simulink model "uz_codegen"  (R2021a)
settings: Solver=VariableStepAuto  StartTime=0.0  StopTime=0.5  RelTol=1e-3  EnableMultiTasking=on
PreLoadFcn:
  | uz_setCodegenPaths
model workspace (MATLAB code in the model file):
  | cmdLim = Simulink.Parameter;
  | cmdLim.Value = 15;
  | cmdLim.Description = 'Limit for controlling the maximum surface command angle.';
  | cmdLim.Min = 0;
  | cmdLim.Max = 90;
  | cmdLim.DocUnits = 'deg';
  | 
  | dispGain = Simulink.Parameter;
  | dispGain.Value = 0.75;
  | dispGain.Description = 'Gain applied to the displacement error.';
  | dispGain.Min = 0;
  | dispGain.Max = [];
  | dispGain.DocUnits = 'deg/sec/deg';
  | 
  | dispLim = Simulink.Parameter;
  | dispLim.Value = 30;
  | dispLim.Description = 'Limit for controlling the maximum commanded angle.';
  | dispLim.Min = 0;
  | dispLim.Max = 180;
  | dispLim.DocUnits = 'deg';
  | 
  | intGain = Simulink.Parameter;
  | intGain.Value = 0.5;
  | intGain.Description = 'Gain applied to the integral error.';
  | intGain.Min = 0;
  | intGain.Max = [];
  | intGain.DocUnits = 'deg/sec/deg/sec';
  | 
  | intLim = Simulink.Parameter;
  | intLim.Value = 5;
  | intLim.Description = 'Limit for controlling the maximum commanded angle.';
  | intLim.Min = 0;
  | intLim.Max = 90;
  | intLim.DocUnits = 'deg';
  | 
  | rateGain = Simulink.Parameter;
  | rateGain.Value = 2;
  | rateGain.Description = 'Gain applied to the rate error.';
  | rateGain.Min = 0;
  | rateGain.Max = [];
  | rateGain.DocUnits = 'deg/deg/sec';
  | 
  | rateLim = Simulink.Parameter;
  | rateLim.Value = 6;
  | rateLim.Description = 'Limit for controlling the maximum commanded angle.';
  | rateLim.Min = 0;
  | rateLim.Max = 180;
  | rateLim.DocUnits = 'deg/sec';
  | 
  | hdgGain = Simulink.Parameter;
  | hdgGain.Value = 0.015;
values from neighbouring files (symbols this model uses):
  f_switchingInverter = 10000    [PMSM_01_Parameter.m]
  I_max = 50    [PMSM_01_Parameter.m]
  Ki_IdController = Kp_IdController * Ki_IdController    (= 100.530964915)    [PMSM_01_Parameter.m]
  Ki_IqController = Kp_IqController * Ki_IqController    (= 100.530964915)    [PMSM_01_Parameter.m]
  Ki_SpeedController = Kp_SpeedController * Ki_SpeedController    (= 50.6340660401)    [PMSM_01_Parameter.m]
  Kp_IdController = Kp_IdController    (= 0.0402123859659)    [PMSM_01_Parameter.m]
  Kp_IqController = Kp_IqController    (= 0.0402123859659)    [PMSM_01_Parameter.m]
  Kp_SpeedController = Kp_SpeedController    (= 0.725279570921)    [PMSM_01_Parameter.m]
  Ld = Lq    (= 1.6e-05)    [PMSM_01_Parameter.m]
  Lq = 16e-6    (= 1.6e-05)    [PMSM_01_Parameter.m]
  psi_pm = 0.0048    [PMSM_01_Parameter.m]
  T_controller = 1/f_CurrentController    (= 5e-05)    [PMSM_01_Parameter.m]
  T_dead = 2e-6    (= 2e-06)    [PMSM_01_Parameter.m]
  U_DC = 46    [PMSM_01_Parameter.m]
  zp = 21    [PMSM_01_Parameter.m]
undefined symbols (not defined in the file or in its folder): DiscIntNeverNeededParam, U_maxDQ
libraries: nesl_utility x17, ee_lib x15, fl_lib x13, simulink x7, pid_lib x3, dspsrcs4 x3, spsTriangleGeneratorLib x1, spsabctodq0Lib x1, spsdq0toabcLib x1, spsdq0toAlphaBetaZeroLib x1, embmathops x1
(part 1 of 2)
settings Model: RequirementInfo={} %GIDa_fe9045fd_0412_4b6e_8206_617cc20e6fde  FPTRunName=Active  Creator=ts  LastModifiedBy=wilflingti66489
settings SolverCC: AlgebraicLoopSolver=TrustRegion  PositivePriorityOrder=on  AutoInsertRateTranBlk=on
settings DataIOCC: SaveOutput=off  SignalLogging=off  DSMLogging=off  SaveTime=off
settings OptimizationCC: DefaultParameterBehavior=Inlined  UseDivisionForNetSlopeComputation=on  GainParamInheritBuiltInType=on  UseFloatMulNetSlope=on  DefaultUnderspecifiedDataType=single  UseSpecifiedMinMax=on  InlineInvariantSignals=on  PassReuseOutputArgsAs=Individual arguments  NoFixptDivByZeroProtection=on  EfficientFloat2IntCast=on  LifeSpan=1  MaxStackSize=64  OptimizeBlockOrder=speed  DifferentSizesBufferReuse=on  EfficientTunableParamExpr=on
settings DebuggingCC: AllowSymbolicDim=off  SFUnexpectedBacktrackingDiag=warning  SFNoUnconditionalDefaultTransitionDiag=warning  SFExecutionAtInitializationDiag=none  SFMachineParentedDataDiag=warning  ArithmeticOperatorsInVariantConditions=warning
settings HardwareCC: ProdBitPerPointer=32  ProdBitPerSizeT=32  ProdBitPerPtrDiffT=32  ProdLargestAtomicInteger=Long  ProdLargestAtomicFloat=Double  ProdWordSize=32  ProdLongLongMode=on  ProdHWDeviceType=ARM Compatible->ARM Cortex-R  HardwareBoardFeatureSet=SoCBlockset
settings SFSimCC: MATLABDynamicMemAlloc=off
settings RTWCC: SystemTargetFile=ert.tlc  GenCodeOnly=on  TemplateMakefile=ert_default_tmf  GenerateReport=on  BuildConfiguration=Faster Runs  IncludeHyperlinkInReport=on  GenerateCodeMetricsReport=on  CheckMdlBeforeBuild=Warning
settings CodeAppCC: ForceParamTrailComments=on  IgnoreCustomStorageClasses=off  OperatorAnnotations=on  SimulinkDataObjDesc=on  SFDataObjDesc=on  MATLABFcnDesc=on  CustomSymbolStrGlobalVar=rt$N$M  CustomSymbolStrType=$N$M  CustomSymbolStrFcn=$N$M$F  CustomSymbolStrMacro=$N$M  InsertBlockDesc=on  StateflowObjectComments=on  MATLABSourceComments=on  EnableCustomComments=on  ReqsInCode=on
settings ERTTargetCC: TargetLangStandard=C99 (ISO)  CodeReplacementLibrary=GNU C99 extensions  MultiwordLength=2048  IncludeMdlTerminateFcn=off  CombineSignalStateStructs=on  SuppressErrorStatus=on  IncludeFileDelimiter=UseQuote  CodeInterfacePackaging=Reusable function  RemoveResetFunc=off  InlinedParameterPlacement=NonHierarchical  MultiInstanceErrorCode=Warning  RootIOFormat=Part of model data structure  ERTCustomFileTemplate=example_file_process.tlc  GlobalDataDefinition=InSourceFile  GlobalDataReference=InSourceFile  ERTFilePackagingFormat=CompactWithDataFile
settings ConfigComp: CovScope=ReferencedModels  CovSaveName=covdata_rollAP  CovMetricSettings=dcmtrwe  CovHTMLOptions=-sRT=1 -aTS=1 -bRG=1 -bTC=1 -hTR=1 -nFC=0 -scm=1 -bcm=1 -xEv=0  CovSaveCumulativeToWorkspaceVar=on  CovSaveSingleToWorkspaceVar=on  CovCumulativeVarName=covCumulativeData_rollAP  CovReportOnPause=off  CovExternalEMLEnable=off  CovSFcnEnable=off

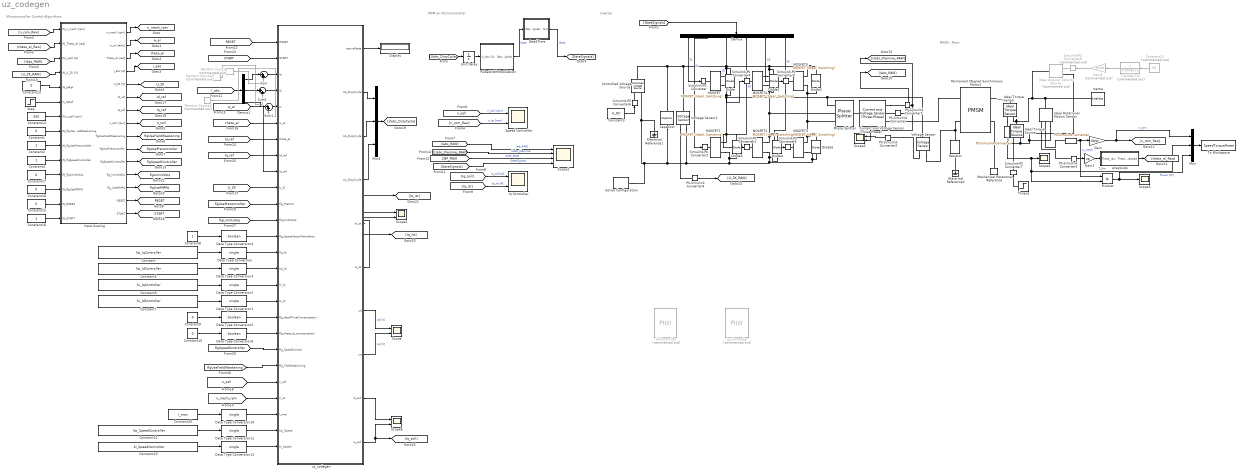
== system uz_codegen ==
  note: Inverter
  note: PWM on Microcontroller
  note: PMSM - Plant
  note: Microcontroller Control-Algorithms
  " " : nesl_utility/PS-Simulink Converter  PhysicalDomain=network_engine_domain  SubClassName=ps_output  LeftPortType=input  RightPortType=output  PseudoPeriodic=off  Frequencies=[]  Unit=inherit  AffineConversion=off
      settings: SourceProductBaseCode=PW,SS
  " 1" : nesl_utility/PS-Simulink Converter  PhysicalDomain=network_engine_domain  SubClassName=ps_output  LeftPortType=input  RightPortType=output  PseudoPeriodic=off  Frequencies=[]  Unit=inherit  AffineConversion=off
      settings: SourceProductBaseCode=PW,SS
  Capacitor : fl_lib/Electrical/Electrical Elements/Capacitor  c=Capacitance_CircuitCondensator uF  r=1e-6 Ohm  g=0 1/Ohm  i_specify=off  i_priority=None  i=0 A  i_nominal_specify=off  i_nominal_unit=A  i_nominal_value=1  v_specify=off  v_priority=None  v=0 V  v_nominal_specify=off  v_nominal_unit=V  v_nominal_value=1  vc_specify=off  vc_priority=High  vc=0 V  vc_nominal_specify=off  vc_nominal_unit=V  vc_nominal_value=1
  Constant : Constant  Value=Kp_IqController
  Constant{1,9..10,13,15,17..18} (7 alike) : Constant  Value=0
  Constant12 : Constant  Commented=on  Value=50
  Constant14 : Constant  Value=500
  Constant{2,4,8,16} (4 alike) : Constant
  Constant20 : Constant  Value=I_max
  Constant22 : Constant  Value=Kp_SpeedController
  Constant23 : Constant  Value=Ki_SpeedController
  Constant3 : Constant  Value=U_DC
  Constant5 : Constant  Value=Kp_IdController
  Constant6 : Constant  Value=Ki_IqController
  Constant7 : Constant  Value=Ki_IdController
  Controlled Voltage Source : fl_lib/Electrical/Electrical Sources/Controlled Voltage Source
  Current and Voltage Sensor (Three-Phase) : ee_lib/Sensors & Transducers/Current and Voltage Sensor (Three-Phase)  vMeasurementType=ee.enum.vmeasurement.ll  outputUnit=ee.enum.unit.si  SRated=100e6 V*A  VRated=24e3 V  I_specify=off  I_priority=None  I=[ 0 0 0 ] A  I_nominal_specify=off  I_nominal_unit=A  I_nominal_value=1  V_specify=off  V_priority=None  V=[ 0 0 0 ] V  V_nominal_specify=off  V_nominal_unit=V  V_nominal_value=1
      settings: SourceProductBaseCode=PS  InternalSimscapePortConfiguration="{\"Bottom\":[],\"Left\":[{\"id\":\"N1\",\"label\":\"~1\",\"type\":\"foundation.electrical.three_phase\"}],\"Right\":[{\"id\":\"V_output\",\"label\":\"V\",\"type\":\"output\"},{\"id\":\"I_output\",\"label\":\"I\",\"type\":\"output\"},{\"id\":\"N2\",\"label\":\"~2\",\"type\":\"foundation.electrical.three_phase\"}],\"Top\":[]}"
  Data Type Conversion{,1..3,10..12} (7 alike) : DataTypeConversion  OutDataTypeStr=single
  Data Type Conversion4 : DataTypeConversion  OutDataTypeStr=boolean
  Data Type Conversion5 : DataTypeConversion  OutDataTypeStr=boolean
  Data Type Conversion6 : DataTypeConversion  OutDataTypeStr=boolean
  DeadTime : Subsystem
  Demux : Demux  Outputs=6
  Demux1 : Demux  Outputs=3
  Diode{,1..5} (6 alike) : ee_lib/Semiconductors & Converters/Diode  ModelType=ee.enum.diode.modelType.pwl  IfMat=[.07, .12, .19, 1.75, 4.24, 7.32, 11.2; .16, .3, .72, 2.14, 4.02, 6.35, 9.12] A  TjVec=[25, 125] degC  VfVec=[.5, .7, .9, 1.3, 1.7, 2.1, 2.5] V  Vf=0.1 V  Ron=0.001 Ohm  Goff=1e-5 1/Ohm  prmExp=ee.enum.diode.expParam.useTwo  I12=[.0137, .545] A  V12=[.6, .7] V  IS=1e-12 A  ec=1  I1=0.0137 A  V1=0.6 V  RS=0 Ohm  Tmeas=25 degC  N_series=1  N_parallel=1  Rz=0.3 Ohm  BV=inf V  C_param=ee.enum.diode.capParam.fixed  CJ=0 pF  CJ0=5 pF  VJ=1 V  Mgrad=0.5  Vvec=[.1, 10, 100] V  Cvec=[3.5, 1, .4] pF  FC=0.5  Q_param=ee.enum.diode.recoveryParam.off  iRM=-7.15 A  iF=4 A  didt=-750 A/us  trr_factor=3  trr=115 ns  Qrr=1500 s*uA  TT=50 ns  tau=100 ns  T_param=ee.enum.diode.temperatureParam.off  IS_T2=1.25e-7 A  I1_T2=0.245 A  V1_T2=0.5 V  Tmeas2=125 degC  EG_param=ee.enum.diode.egapParam.material_si  EG=1.11 eV  XTI_param=ee.enum.diode.xtiParam.pn  XTI=3  dBVdT=0 V/K  enable_faults=ee.enum.faults.faultEnable.no  fault_action=ee.enum.faults.faultAction.none  fault_types=ee.enum.diode.faults.open  tau_fault=1e-3 s  IfMat_faulted=[.07, .12, .19, 1.75, 4.24, 7.32, 11.2; .16, .3, .72, 2.14, 4.02, 6.35, 9.12] A  VfVec_faulted=[.5, .7, .9, 1.3, 1.7, 2.1, 2.5] V  Ropen_faulted=1000 Ohm  Gshort_faulted=1000 1/Ohm  Vf_faulted=0.6 V  Ron_faulted=0.3 Ohm  Goff_faulted=1e-8 S  I12_faulted=[.0137, .545] A  V12_faulted=[.6, .7] V  IS_faulted=1e-12 A  ec_faulted=1  I1_faulted=0.0137 A  V1_faulted=0.6 V  RS_faulted=0 Ohm  Rz_faulted=0.3 Ohm  BV_faulted=inf V  Cscale_faulted=100  enable_temporal_fault=ee.enum.faults.faultEnable.no  t_fault=inf s  enable_behavioral_fault=ee.enum.faults.faultEnable.no  max_permissible_voltage=inf V  n_fail_on_voltage=1  max_permissible_current=inf A  t_fail_on_current=1 s  max_permissible_dVdt=inf V/s  Tdevice=25 degC  i_specify=off  i_priority=None  i=0 A  i_nominal_specify=off  i_nominal_unit=A  i_nominal_value=1  v_specify=off  v_priority=None  v=0 V  v_nominal_specify=off  v_nominal_unit=V  v_nominal_value=1  i_diode_specify=off  i_diode_priority=None  i_diode=0 A  i_diode_nominal_specify=off  i_diode_nominal_unit=A  i_diode_nominal_value=1  v_diode_specify=off  v_diode_priority=None  v_diode=0 V  v_diode_nominal_specify=off  v_diode_nominal_unit=V  v_diode_nominal_value=1  i_capacitor_specify=off  i_capacitor_priority=None  i_capacitor=0 A  i_capacitor_nominal_specify=off  i_capacitor_nominal_unit=A  i_capacitor_nominal_value=1  v_capacitor_specify=off  v_capacitor_priority=None  v_capacitor=0 V  v_capacitor_nominal_specify=off  v_capacitor_nominal_unit=V  v_capacitor_nominal_value=1  power_dissipated_specify=off  power_dissipated_priority=None  power_dissipated=0 W  power_dissipated_nominal_specify=off  power_dissipated_nominal_unit=W  power_dissipated_nominal_value=1  max_permissible_temperature=inf K  t_fail_on_temperature=1 s  thermal_network_parameterization=ee.enum.thermalNetworkTopology.cauer  Rth=[0, 10] K/W  Rth_Foster=[4, 6] K/W  thermal_mass_parameterization=ee.enum.thermalNetwork.timeconstant  thermal_mass=[0, 1] J/K  thermal_mass_Foster=[1.5, 3] J/K  thermal_time_constant=[0, 10] s  thermal_time_constant_Foster=[6, 18] s  thermal_mass_initial_temperatures=[25, 25] degC
  Display : Display
  Electrical Reference1 : fl_lib/Electrical/Electrical Elements/Electrical Reference
  Electrical Reference2 : fl_lib/Electrical/Electrical Elements/Electrical Reference
  Gain : Gain  Gain=30/pi
  Gain1 : Gain  Gain=zp
  Gain2 : Gain  Commented=on  Gain=pi/30
  Id-Controller : pid_lib/PID Controller  Commented=on  Controller=PI  Form=Parallel  TimeDomain=Discrete-time  UseExternalTs=off  SampleTime=-1  IntegratorMethod=Forward Euler  FilterMethod=Forward Euler  ControllerParametersSource=external  P=Kp_IqController  I=Ki_IqController  D=0  UseFilter=on  N=100  TunerSelectOption=Transfer Function Based (PID Tuner App)  InitialConditionSource=internal  InitialConditionForIntegrator=0  InitialConditionForFilter=0  DifferentiatorICPrevScaledInput=0  ExternalReset=level  TrackingMode=off  Kt=1  LimitOutput=on  SatLimitsSource=external  UpperSaturationLimit=U_maxDQ  LowerSaturationLimit=-U_maxDQ  LinearizeAsGain=on  AntiWindupMode=none  Kb=1  POutMin=[]  POutMax=[]  IOutMin=[]  IOutMax=[]  DOutMin=[]  DOutMax=[]  NOutMin=[]  NOutMax=[]  SumOutMin=[]  SumOutMax=[]  SaturationOutMin=[]  SaturationOutMax=[]  PParamMin=[]  PParamMax=[]  IParamMin=[]  IParamMax=[]  DParamMin=[]  DParamMax=[]  NParamMin=[]  NParamMax=[]  KbParamMin=[]  KbParamMax=[]  KtParamMin=[]  KtParamMax=[]  KbOutMin=[]  KbOutMax=[]  KtOutMin=[]  KtOutMax=[]  IntegratorOutMin=[]  IntegratorOutMax=[]  FilterOutMin=[]  FilterOutMax=[]  SumI1OutMin=[]  SumI1OutMax=[]  SumI2OutMin=[]  SumI2OutMax=[]  SumI3OutMin=[]  SumI3OutMax=[]  SumI4OutMin=[]  SumI4OutMax=[]  SumDOutMin=[]  SumDOutMax=[]  DifferentiatorOutMin=[]  DifferentiatorOutMax=[]  FilterDiffOutCoefMin=[]  FilterDiffOutCoefMax=[]  ReciprocalOutMin=[]  ReciprocalOutMax=[]  SumDenOutMin=[]  SumDenOutMax=[]  SumNumOutMin=[]  SumNumOutMax=[]  DivideOutMin=[]  DivideOutMax=[]  UdiffTsProdOutMin=[]  UdiffTsProdOutMax=[]  NTsProdOutMin=[]  NTsProdOutMax=[]  UintegralTsProdOutMin=[]  UintegralTsProdOutMax=[]  UngainTsProdOutMin=[]  UngainTsProdOutMax=[]  IntegratorContinuousStateAttributes=''  IntegratorStateMustResolveToSignalObject=off  IntegratorRTWStateStorageClass=Auto  FilterContinuousStateAttributes=''  FilterStateMustResolveToSignalObject=off  FilterRTWStateStorageClass=Auto  ParallelPVariant=ExternalParameters  IdealPVariant=Disabled  IVariant=ExternalParameters  DVariant=Disabled  IntegratorVariant=Discrete  SatVariant=External  AWVariant=Passthrough  PCopyVariant=Disabled  TRVariant=Disabled  FdbkBlocksVariant=Forward  IdealPFdbkVariant=Disabled  SatFdbkVariant=Disabled  DerivativeFilterVariant=Disabled  NVariant=Disabled  NCopyVariant=Disabled_SignalSpec  FilterICVariant=Disabled  IntegratorICVariant=InternalICs  ExternalResetVariant=ExternalReset  TRSumVariant=Passthrough  SumFdbkVariant=Disabled  SumVariant=Sum_PI  TsampFilterVariant=InternalTs  TsampNgainVariant=Passthrough  TsampIntegralVariant=Passthrough  ExternalSaturationOutDataTypeStr=Inherit: Same as second input
  Ideal Angular Velocity Source : fl_lib/Mechanical/Mechanical Sources/Ideal Angular Velocity Source  Commented=on
  Ideal Rotational Motion Sensor : fl_lib/Mechanical/Mechanical Sensors/Ideal Rotational Motion Sensor  wrap_angle=simscape.enum.onoff.on  offset=0 rad
  Ideal Torque Sensor : fl_lib/Mechanical/Mechanical Sensors/Ideal Torque Sensor
  Ideal Torque Source : fl_lib/Mechanical/Mechanical Sources/Ideal Torque Source
  Inertia : fl_lib/Mechanical/Rotational Elements/Inertia  inertia=J_M kg*m^2  num_ports=foundation.enum.numPorts2.one  w_specify=off  w_priority=High  w=0 rad/s  w_nominal_specify=off  w_nominal_unit=rad/s  w_nominal_value=1  t_specify=off  t_priority=None  t=0 N*m  t_nominal_specify=off  t_nominal_unit=N*m  t_nominal_value=1
  Input Scaling : Subsystem
  Iq Controller : Scope  NumInputPorts=2
  Iq_Controller : pid_lib/PID Controller  Commented=on  Controller=PI  Form=Parallel  TimeDomain=Discrete-time  UseExternalTs=off  SampleTime=-1  IntegratorMethod=Forward Euler  FilterMethod=Forward Euler  ControllerParametersSource=external  P=Kp_IqController  I=Ki_IqController  D=0  UseFilter=on  N=100  TunerSelectOption=Transfer Function Based (PID Tuner App)  InitialConditionSource=internal  InitialConditionForIntegrator=0  InitialConditionForFilter=0  DifferentiatorICPrevScaledInput=0  ExternalReset=level  TrackingMode=off  Kt=1  LimitOutput=on  SatLimitsSource=external  UpperSaturationLimit=U_maxDQ  LowerSaturationLimit=-U_maxDQ  LinearizeAsGain=on  AntiWindupMode=none  Kb=1  POutMin=[]  POutMax=[]  IOutMin=[]  IOutMax=[]  DOutMin=[]  DOutMax=[]  NOutMin=[]  NOutMax=[]  SumOutMin=[]  SumOutMax=[]  SaturationOutMin=[]  SaturationOutMax=[]  PParamMin=[]  PParamMax=[]  IParamMin=[]  IParamMax=[]  DParamMin=[]  DParamMax=[]  NParamMin=[]  NParamMax=[]  KbParamMin=[]  KbParamMax=[]  KtParamMin=[]  KtParamMax=[]  KbOutMin=[]  KbOutMax=[]  KtOutMin=[]  KtOutMax=[]  IntegratorOutMin=[]  IntegratorOutMax=[]  FilterOutMin=[]  FilterOutMax=[]  SumI1OutMin=[]  SumI1OutMax=[]  SumI2OutMin=[]  SumI2OutMax=[]  SumI3OutMin=[]  SumI3OutMax=[]  SumI4OutMin=[]  SumI4OutMax=[]  SumDOutMin=[]  SumDOutMax=[]  DifferentiatorOutMin=[]  DifferentiatorOutMax=[]  FilterDiffOutCoefMin=[]  FilterDiffOutCoefMax=[]  ReciprocalOutMin=[]  ReciprocalOutMax=[]  SumDenOutMin=[]  SumDenOutMax=[]  SumNumOutMin=[]  SumNumOutMax=[]  DivideOutMin=[]  DivideOutMax=[]  UdiffTsProdOutMin=[]  UdiffTsProdOutMax=[]  NTsProdOutMin=[]  NTsProdOutMax=[]  UintegralTsProdOutMin=[]  UintegralTsProdOutMax=[]  UngainTsProdOutMin=[]  UngainTsProdOutMax=[]  IntegratorContinuousStateAttributes=''  IntegratorStateMustResolveToSignalObject=off  IntegratorRTWStateStorageClass=Auto  FilterContinuousStateAttributes=''  FilterStateMustResolveToSignalObject=off  FilterRTWStateStorageClass=Auto  ParallelPVariant=ExternalParameters  IdealPVariant=Disabled  IVariant=ExternalParameters  DVariant=Disabled  IntegratorVariant=Discrete  SatVariant=External  AWVariant=Passthrough  PCopyVariant=Disabled  TRVariant=Disabled  FdbkBlocksVariant=Forward  IdealPFdbkVariant=Disabled  SatFdbkVariant=Disabled  DerivativeFilterVariant=Disabled  NVariant=Disabled  NCopyVariant=Disabled_SignalSpec  FilterICVariant=Disabled  IntegratorICVariant=InternalICs  ExternalResetVariant=ExternalReset  TRSumVariant=Passthrough  SumFdbkVariant=Disabled  SumVariant=Sum_PI  TsampFilterVariant=InternalTs  TsampNgainVariant=Passthrough  TsampIntegralVariant=Passthrough  ExternalSaturationOutDataTypeStr=Inherit: Same as second input
  MOSFET{,1..5} (6 alike) : ee_lib/Semiconductors & Converters/MOSFET (Ideal, Switching)  Rds=0.040 Ohm  Goff=1e-6 1/Ohm  Vth=0.7 V  diode_param=1  diode_Vf=0.8 V  diode_Ron=0.001 Ohm  diode_Goff=1e-5 1/Ohm  diode_C=5e-8 F  diode_iRM=-235 A  diode_iF=300 A  diode_idot=-50 A/us  diode_trr_param=1  diode_trr_factor=3  diode_trr=15 us  diode_Qrr=1.5e+3 s*uA  thermal_loss_option=ee.enum.converters.thermalLossOption.constantvalues  Von_data=[0, 1.1, 1.3, 1.45, 1.75, 2.25, 2.7; 0, 1, 1.15, 1.35, 1.7, 2.35, 3] V  Eon_data=[0, .29, 1.43, 2.86, 5.71, 13.14, 22.86; 0, .57, 2.63, 5.14, 10.29, 20.57, 30.29] * 1e-3 J  Eoff_data=[0, .21, 1.07, 2.14, 4.29, 9.86, 17.14; 0, .43, 1.97, 3.86, 7.71, 15.43, 22.71] * 1e-3 J  Tj=[298.15, 398.15] K  Iout_data=[0, 10, 50, 100, 200, 400, 600] A  Eon_scalar=22.86e-3 J  Eoff_scalar=17.14e-3 J  Voff=300 V  Iout_scalar=600 A  diodeModelType=ee.enum.converters.diodeModelType.pwl  diode_IfMat=[.07, .12, .19, 1.75, 4.24, 7.32, 11.2; .16, .3, .72, 2.14, 4.02, 6.35, 9.12] A  diode_TjVec=[25, 125] degC  diode_VfVec=[.5, .7, .9, 1.3, 1.7, 2.1, 2.5] V  thermal_network_parameterization=ee.enum.thermalNetworkTopology.external  Rth=[.03, .2] K/W  Rth_Foster=[.03, .2] K/W  thermal_mass_parameterization=ee.enum.thermalNetwork.timeconstant  thermal_mass=[3, 25] J/K  thermal_mass_Foster=[33, 50] J/K  thermal_time_constant=[.1, 5] s  thermal_time_constant_Foster=[1, 10] s  thermal_mass_initial_temperatures=[25, 25] degC  junction_thermal_mass=0.1 J/K  vT_specify=off  vT_priority=None  vT=0 V  vT_nominal_specify=off  vT_nominal_unit=V  vT_nominal_value=1  Qj_specify=off  Qj_priority=None  Qj=0 W  Qj_nominal_specify=off  Qj_nominal_unit=W  Qj_nominal_value=1  junction_temperature_specify=off  junction_temperature_priority=None  junction_temperature=25 degC  junction_temperature_nominal_specify=off  junction_temperature_nominal_unit=degC  junction_temperature_nominal_value=1
  Mechanical Rotational Reference : fl_lib/Mechanical/Rotational Elements/Mechanical Rotational Reference
  Mux : Mux  Inputs=3
  Mux1 : Mux  Inputs=3
  PS-Simulink Converter{,1..4} (5 alike) : nesl_utility/PS-Simulink Converter  PhysicalDomain=network_engine_domain  SubClassName=ps_output  LeftPortType=input  RightPortType=output  PseudoPeriodic=off  Frequencies=[]  Unit=inherit  AffineConversion=off
      settings: SourceProductBaseCode=PW,SS
  Permanent Magnet Synchronous Motor1 : ee_lib/Electromechanical/Permanent Magnet/PMSM  winding_type=ee.enum.statorconnection.wye  machine_param=ee.enum.pmsm.parameterization.constant  nPolePairs=zp  pmflux_param=ee.enum.pmflux.fluxlinkage  pm_flux_linkage=psi_pm Wb  torque_constant=0.18 N*m/A  back_emf_constant=0.07 V/(rad/s)  stator_param=ee.enum.statorparam.LdLqL0  Ld=Ld H  Lq=Lq H  idVec=[-200, 0, 200] A  iqVec=[-200, 0, 200] A  LdMatrix=0.0002 * ones(3, 3) H  LqMatrix=0.0002 * ones(3, 3) H  PmMatrix=0.1 * ones(3, 3) Wb  ktMatrix=0.18 * ones(3, 3) N*m/A  keMatrix=0.18 * ones(3, 3) V/(rad/s)  L0=0.00016 H  Ls=0.0002 H  Lm=-0.00002 H  Ms=0.00002 H  Rs=R Ohm  zero_sequence=ee.enum.park.zerosequence.include  J=0.0 kg*m^2  lam=0 N*m/(rad/s)  axes_param=ee.enum.rotorangle.daxis  i_d_specify=off  i_d_priority=None  i_d=0 A  i_d_nominal_specify=off  i_d_nominal_unit=A  i_d_nominal_value=1  i_q_specify=off  i_q_priority=None  i_q=0 A  i_q_nominal_specify=off  i_q_nominal_unit=A  i_q_nominal_value=1  torque_specify=off  torque_priority=None  torque=0 N*m  torque_nominal_specify=off  torque_nominal_unit=N*m  torque_nominal_value=1  angular_velocity_specify=off  angular_velocity_priority=High  angular_velocity=0 deg/s  angular_velocity_nominal_specify=off  angular_velocity_nominal_unit=rpm  angular_velocity_nominal_value=1  angular_position_specify=off  angular_position_priority=High  angular_position=0 deg  angular_position_nominal_specify=off  angular_position_nominal_unit=deg  angular_position_nominal_value=1  loss_param=ee.enum.ironloss.none  losses_oc=[0, 0, 0] W  losses_sc=[0, 0, 0] W  f_losses=60 Hz  Isc_losses=95 A  Tmeas=298.15 K  alpha=3.93e-3 1/K  alpha_flux=-0.001 1/K  stator_thermal_mass=100 J/K  rotor_thermal_mass=200 J/K  Rm_percent_rotor=90  Rd_percent_rotor=30  temperatureA_specify=off  temperatureA_priority=High  temperatureA=25 degC  temperatureA_nominal_specify=off  temperatureA_nominal_unit=degC  temperatureA_nominal_value=1  temperatureB_specify=off  temperatureB_priority=High  temperatureB=25 degC  temperatureB_nominal_specify=off  temperatureB_nominal_unit=degC  temperatureB_nominal_value=1  temperatureC_specify=off  temperatureC_priority=High  temperatureC=25 degC  temperatureC_nominal_specify=off  temperatureC_nominal_unit=degC  temperatureC_nominal_value=1  temperatureR_specify=off  temperatureR_priority=High  temperatureR=25 degC  temperatureR_nominal_specify=off  temperatureR_nominal_unit=degC  temperatureR_nominal_value=1
      settings: InternalSimscapePortConfiguration="{\"Bottom\":[],\"Left\":[{\"id\":\"N\",\"label\":\"~\",\"type\":\"foundation.electrical.three_phase\"},{\"id\":\"n\",\"label\":\"n\",\"type\":\"foundation.electrical.electrical\"}],\"Right\":[{\"id\":\"R\",\"label\":\"R\",\"type\":\"foundation.mechanical.rotational.rotational\"},{\"id\":\"C\",\"label\":\"C\",\"type\":\"foundation.mechanical.rotational.rotational\"}],\"Top\":[]}"
  Phase Splitter : ee_lib/Connectors & References/Phase Splitter
      settings: SourceProductBaseCode=PS
  Product : Product
  PulseWidthModulation : Subsystem
  Random Source : dspsrcs4/Random Source  Commented=on  SrcType=Uniform  NormMethod=Ziggurat  CltLength=12  MinVal=-0.5  MaxVal=0.5  MeanVal=0  VarVal=1  RepMode=Not repeatable  rawSeed=1  IsInherit=off  SampMode=Discrete  SampTime=T_controller  SampFrame=1  DataType=Single  OutComplex=Real  OutputFrames=off
  Random Source1 : dspsrcs4/Random Source  Commented=on  SrcType=Uniform  NormMethod=Ziggurat  CltLength=12  MinVal=-0.5  MaxVal=0.5  MeanVal=0  VarVal=1  RepMode=Not repeatable  rawSeed=1  IsInherit=off  SampMode=Discrete  SampTime=T_controller  SampFrame=1  DataType=Single  OutComplex=Real  OutputFrames=off
  Random Source2 : dspsrcs4/Random Source  Commented=on  SrcType=Uniform  NormMethod=Ziggurat  CltLength=12  MinVal=-0.5  MaxVal=0.5  MeanVal=0  VarVal=1  RepMode=Not repeatable  rawSeed=1  IsInherit=off  SampMode=Discrete  SampTime=T_controller  SampFrame=1  DataType=Single  OutComplex=Real  OutputFrames=off
  Resistor : fl_lib/Electrical/Electrical Elements/Resistor  R=2000 Ohm  i_specify=off  i_priority=None  i=0 A  i_nominal_specify=off  i_nominal_unit=A  i_nominal_value=1  v_specify=off  v_priority=None  v=0 V  v_nominal_specify=off  v_nominal_unit=V  v_nominal_value=1
  Scope{,1,3,6} (4 alike) : Scope  NumInputPorts=2
  Scope2 : Scope  NumInputPorts=4
  Scope4 : Scope
  Scope5 : Scope
  Simulink-PS Converter{,1..7} (8 alike) : nesl_utility/Simulink-PS Converter  PhysicalDomain=network_engine_domain  SubClassName=ps_input  LeftPortType=input  RightPortType=output  PseudoPeriodic=off  Frequencies=[]  NoiseDistribution=none  NoiseParameters=[]  Unit=1  AffineConversion=off  FilteringAndDerivatives=provide  SimscapeFilterOrder=1  InputFilterTimeConstant=0.001  UdotUserProvided=0
      settings: SourceProductBaseCode=PW,SS
  Simulink-PS Converter9 : nesl_utility/Simulink-PS Converter  Commented=on  PhysicalDomain=network_engine_domain  SubClassName=ps_input  LeftPortType=input  RightPortType=output  PseudoPeriodic=off  Frequencies=[]  NoiseDistribution=none  NoiseParameters=[]  Unit=1  AffineConversion=off  FilteringAndDerivatives=filter  SimscapeFilterOrder=1  InputFilterTimeConstant=0.001  UdotUserProvided=0
      settings: SourceProductBaseCode=PW,SS
  Solver Configuration : nesl_utility/Solver Configuration  PhysicalDomain=network_engine_domain  SubClassName=solver  LeftPortType=input  RightPortType=generic  Tones=[]  Harmonics=[]  SimulateNoise=off  Profile=off  UseLocalSampling=off  EnableSwitchedLinearOptims=on  FrequencyDomain=off  UseCCode=off  RelTol=0.001  AbsTol=1e-06  MinStep=1e-09  ToWorkspace=off  RevertToSquareIcSolve=off  NumHomotopyIterations=100  PhasorMode=off  PhasorModeNumHarmonics=1  DoDC=off  ResidualTolerance=1e-09  UseLocalSolver=off  LocalSolverChoice=NE_BACKWARD_EULER_ADVANCER  LocalSolverSampleTime=0.001  DoFixedCost=off  MaxNonlinIter=3  MaxModeIter=2  ComputeImpulses=off  ImpulseIterations=2  LinearAlgebra=auto  EquationFormulation=NE_TIME_EF  DelaysMemoryBudget=1024  AutomaticFiltering=on  FilteringTimeConstant=0.001  PartitionStorageMethod=AS_NEEDED  PartitionMemoryBudget=1024  PartitionMethod=ROBUST
      settings: SourceProductBaseCode=PW,SS
  Speed Controller : Scope  NumInputPorts=2
  Step : Step  Time=0.02  SampleTime=0
  Sum : Sum  Inputs=|++
  Sum1 : Sum  Inputs=|++
  Sum2 : Sum  Inputs=|++
  To Workspace : ToWorkspace  VariableName=SpeedTorquePower  SaveFormat=Timeseries  SampleTime=-1
  Torque : Step  Time=0.04  After=0  SampleTime=0
  Transfer Fcn : TransferFcn  Commented=on  Denominator=[0.0005 1]
  Unit Delay : UnitDelay  SampleTime=1/f_switchingInverter  HasFrameUpgradeWarning=on
  Voltage Sensor : fl_lib/Electrical/Electrical Sensors/Voltage Sensor
  Voltage Sensor1 : fl_lib/Electrical/Electrical Sensors/Voltage Sensor
  uz_codegen : Stateflow chart  TreatAsAtomicUnit=on
      settings: PortSchema="{\"entries\":[{\"content\":{\"sides\":[{\"content\":{\"connectorIds\":[\"In10\",\"In11\",\"In5\",\"In3\",\"In2\",\"In4\",\"In6\",\"In8\",\"In7\",\"In9\",\"In1\",\"In12\",\"In13\",\"In14\",\"In15\",\"In16\",\"In17\",\"In18\",\"In19\",\"In20\",\"In21\",\"In22\",\"In23\",\"In24\",\"In25\",\"In26\"]},\"type\":\"ConnectorPlacement.EquallySpacedRectSide\",\"uuid\":\"76a4c5fd-8833-454d-a27c-9cb5ddbec7a7\"},{\"content\":{\"connectorIds\":[\"Out2\",\"Out1\",\"Out4\",\"Out3\",\"Out6\",\"Out5\",\"Out8\",\"Out7\",\"Out10\",\"Out9\"],\"side\":\"RIGHT\"},\"type\":\"ConnectorPlacement.EquallySpacedRectSide\",\"uuid\":\"21c8cff2-6555-410e-8e51-882650c7a948\"},{\"content\":{\"connectorIds\":[],\"side\":\"TOP\"},\"type\":\"ConnectorPlacement.EquallySpacedRectSide\",\"uuid\":\"0c75ee88-c520-42c4-9c42-3a1aac3b64b6\"}]},\"type\":\"ConnectorPlacement.EquallySpacedConnector\",\"uuid\":\"5756a7ca-2edf-4f43-a7f7-e1c56b726d1a\"}],\"packageUris\":[\"http://schema.mathworks.com/mf0/Connector/R2020b\"],\"version\":\"1.0\"}"
  wrapto2pi : Subsystem
  tag scope: I_abc=global, Id_ref=global, Iq_ref=global, RESET=global, START=global, U_ZK=global, flgLimitUdUq=global, flgSpeedController=global, flgUseFieldWeakening=global, flgUseMMPA=global, flgUsePrecontroller=global, n_mech_rpm=global, n_soll=global, theta_el=global, w_el=global
  wires:
  PS-Simulink Converter3/1 -> Gain1/1
  PS-Simulink Converter1/1 -> [Uabc_Klemme_RAW], Scope3/2
  Constant10/1 -> Data Type Conversion6/1
  Data Type Conversion6/1 -> uz_codegen/19(flg_theta_el_compensation)
  Demux/1 -> Simulink-PS Converter/1  "S1"
  Product/1 -> Mux/3, Scope5/1  "Power [W]"
  DeadTime/1(Out) -> [GateSignals]  "Gate"
  Data Type Conversion5/1 -> uz_codegen/18(flg_deadTimeCompensation)
  Constant5/1 -> Data Type Conversion3/1
  [U_ZK] -> uz_codegen/9(U_IC)
  Constant14/1 -> Input Scaling/7(IN_n_soll [rpm])
  [theta_el] -> uz_codegen/6(theta_el)
  [Iq_ist] -> Iq Controller/2  "Iq_ist [A]"
  Constant8/1 -> Data Type Conversion4/1
  PulseWidthModulation/1(GateSignals) -> DeadTime/1(GateSignals)  "Gate"
  Input Scaling/7(Iq_ref) -> [Iq_ref]
  wrapto2pi/1(Theta_wrapped) -> [theta_el_Raw]
  Unit Delay/1 -> PulseWidthModulation/1(U_abc [V])
  uz_codegen/5(iq_ist) -> Scope1/2, [Iq_ist]
  Constant2/1 -> Input Scaling/9(IN_flgUsePrecontroller)
  Constant18/1 -> Input Scaling/12(IN_flgUseMMPA)
  Input Scaling/9(flgUseFieldWeakening) -> [flgUseFieldWeakening]
  [Id_ref] -> uz_codegen/8(id_ref)
  Demux1/1 -> Sum/1
  Constant1/1 -> Input Scaling/8(IN_flgUseFieldWeakening)
  [Uabc_DutyCycle] -> Unit Delay/1
  [n_rpm_Raw] -> Speed Controller/2  "n_ist [rpm]"
  Data Type Conversion2/1 -> uz_codegen/16(Ki_Iq)
  Demux1/3 -> Sum1/1
  Gain1/1 -> wrapto2pi/1(Theta_raw)
  [START] -> uz_codegen/11(START)
  [Iabc_RAW] -> Scope2/1  "Iab_RAW"
  Data Type Conversion/1 -> uz_codegen/14(Kp_Iq)
  [flgLimitUdUq] -> uz_codegen/12(flgLimitUdUq)
  Step/1 -> Input Scaling/6(In_IqRef)
  Demux/3 -> Simulink-PS Converter4/1  "S2"
  Constant6/1 -> Data Type Conversion2/1
  Input Scaling/4(I_abc [A]) -> [I_abc]
  Input Scaling/3(Theta_el [rad]) -> [theta_el]
  Constant7/1 -> Data Type Conversion1/1
  Data Type Conversion1/1 -> uz_codegen/17(Ki_Id)
  " "/1 -> Product/1, Gain/1  "w_mech"
  uz_codegen/6(id_ist) -> [Id_ist], Scope1/1
  uz_codegen/2(activeState) -> Display/1
  PS-Simulink Converter/1 -> [Iabc_RAW]
  [n_rpm_Raw] -> Input Scaling/1(IN_n_mech [rpm])
  Constant/1 -> Data Type Conversion/1
  uz_codegen/4(Ub_DutyCycle) -> Mux1/2
  Constant16/1 -> Input Scaling/14(IN_START)
  Input Scaling/2(w_el [rad/s]) -> [w_el]
  Constant15/1 -> Input Scaling/13(IN_RESET)
  Constant17/1 -> Input Scaling/11(IN_flgLimitUdUq)
  uz_codegen/3(Uc_DutyCycle) -> Mux1/3
  Input Scaling/13(flg_UseMMPA) -> [flgUseMMPA]
  " 1"/1 -> Product/2, Mux/2, Scope4/1  "T_Nm"
  Input Scaling/12(flg_LimitUdUq) -> [flgLimitUdUq]
  Transfer Fcn/1 -> Gain2/1
  [w_el] -> uz_codegen/4(w_el)
  Input Scaling/8(n_soll [rpm]) -> [n_soll]
  Input Scaling/11(flgSpeedController) -> [flgSpeedController]
  Input Scaling/6(Id_ref) -> [Id_ref]
  Demux/4 -> Simulink-PS Converter1/1  "S5"
  [flgUsePrecontroller] -> uz_codegen/1(flg_PreCntr)
  [Iabc_RAW] -> Input Scaling/3(IN_I_abc [A])
  Gain2/1 -> Simulink-PS Converter9/1
  [U_ZK_RAW] -> Input Scaling/4(IN_U_ZK [V])
  Demux/5 -> Simulink-PS Converter3/1  "S3"
  Demux/2 -> Simulink-PS Converter2/1  "S4"
  Demux/6 -> Simulink-PS Converter5/1  "S6"
  [Iq_soll] -> Iq Controller/1  "Iq_soll [A]"
  [CMP_PWM] -> Scope2/3  "CMP_PWM"
  Input Scaling/1(n_mech [rpm]) -> [n_mech_rpm]
  Constant12/1 -> Transfer Fcn/1
  Demux1/2 -> Sum2/1
  Input Scaling/5(U_ZK [V]) -> [U_ZK]
  PS-Simulink Converter2/1 -> Scope3/1
  Gain/1 -> Mux/1, [n_rpm_Raw]  "n_rpm"
  Constant3/1 -> Simulink-PS Converter6/1
  Mux1/1 -> [Uabc_DutyCycle]
  uz_codegen/8(ud) -> Scope/1  "Ud [V]"
  [GateSignals] -> Demux/1
  [GateSignals] -> Scope2/4  "GateSignals"
  [RESET] -> uz_codegen/10(RESET)
  uz_codegen/1(Ua_DutyCycle) -> Mux1/1
  Constant9/1 -> Data Type Conversion5/1
  Constant4/1 -> Input Scaling/10(IN_flgSpeedController)
  Input Scaling/15(START) -> [START]
  uz_codegen/7(uq) -> Scope/2  "Uq [V]"
  PS-Simulink Converter4/1 -> [U_ZK_RAW]
  Constant13/1 -> Input Scaling/5(IN_IdRef)
  [Uabc_Klemme_RAW] -> Scope2/2  "Uabc_Klemme"
  Torque/1 -> Simulink-PS Converter7/1
  Mux/1 -> To Workspace/1
  Data Type Conversion4/1 -> uz_codegen/13(flg_SpaceVectorModulation)
  [n_soll] -> Speed Controller/1  "n_soll [rpm]"
  Input Scaling/10(flgUsePrecontroller) -> [flgUsePrecontroller]
  [Iq_ref] -> uz_codegen/7(iq_ref)
  Input Scaling/14(RESET) -> [RESET]
  [theta_el_Raw] -> Input Scaling/2(IN_Theta_el [rad])
  Data Type Conversion3/1 -> uz_codegen/15(Kp_Id)
  [I_abc] -> Demux1/1
  Sum/1 -> uz_codegen/5(ia)
  Sum2/1 -> uz_codegen/3(ib)
  Sum1/1 -> uz_codegen/2(ic)
  Random Source/1 -> Sum/2
  Random Source1/1 -> Sum2/2
  Random Source2/1 -> Sum1/2
  [flgUseFieldWeakening] -> uz_codegen/21(flg_FieldWeakening)
  Constant20/1 -> Data Type Conversion10/1
  Constant22/1 -> Data Type Conversion11/1
  Constant23/1 -> Data Type Conversion12/1
  Data Type Conversion12/1 -> uz_codegen/26(Ki_Speed)
  Data Type Conversion11/1 -> uz_codegen/25(Kp_Speed)
  Data Type Conversion10/1 -> uz_codegen/24(I_max)
  [n_mech_rpm] -> uz_codegen/23(n_ist)
  [n_soll] -> uz_codegen/22(n_ref)
  uz_codegen/9(iq_soll) -> [Iq_soll], Scope6/2
  uz_codegen/10(id_soll) -> Scope6/1
  [flgSpeedController] -> uz_codegen/20(flg_SpeedControl)
  connections:
  Ideal Torque Sensor/RConn1 -- Ideal Torque Source/LConn1 -- Ideal Angular Velocity Source/LConn1 -- Inertia/LConn1 -- Ideal Rotational Motion Sensor/LConn1
  MOSFET3/RConn1 -- MOSFET5/RConn2 -- Diode2/LConn1 -- Phase Splitter/RConn3 -- Diode5/RConn1
  MOSFET2/RConn2 -- MOSFET1/RConn2 -- Diode3/LConn1 -- Solver Configuration/RConn1 -- Electrical Reference1/LConn1 -- Controlled Voltage Source/RConn2 -- Capacitor/RConn1 -- Voltage Sensor1/RConn2 -- Diode5/LConn1 -- MOSFET3/RConn2 -- Diode4/LConn1
  Voltage Sensor/RConn2 -- Permanent Magnet Synchronous Motor1/LConn2 -- Resistor/LConn1
  Ideal Torque Source/RConn2 -- Permanent Magnet Synchronous Motor1/RConn2 -- Mechanical Rotational Reference/LConn1 -- Ideal Angular Velocity Source/RConn2 -- Ideal Rotational Motion Sensor/RConn1
  Diode/LConn1 -- MOSFET1/RConn1 -- Diode3/RConn1 -- Voltage Sensor/LConn1 -- Phase Splitter/RConn1 -- MOSFET/RConn2
  MOSFET2/RConn1 -- Diode4/RConn1 -- MOSFET4/RConn2 -- Diode1/LConn1 -- Phase Splitter/RConn2
  Diode/RConn1 -- MOSFET4/RConn1 -- Diode1/RConn1 -- MOSFET5/RConn1 -- Diode2/RConn1 -- Controlled Voltage Source/LConn1 -- Capacitor/LConn1 -- Voltage Sensor1/LConn1 -- MOSFET/RConn1
  Current and Voltage Sensor (Three-Phase)/RConn1 -- PS-Simulink Converter1/LConn1
  PS-Simulink Converter/LConn1 -- Current and Voltage Sensor (Three-Phase)/RConn2
  Current and Voltage Sensor (Three-Phase)/LConn1 -- Phase Splitter/LConn1
  PS-Simulink Converter3/LConn1 -- Ideal Rotational Motion Sensor/RConn3
  Simulink-PS Converter3/RConn1 -- MOSFET5/LConn1
  MOSFET/LConn1 -- Simulink-PS Converter/RConn1
  Simulink-PS Converter7/RConn1 -- Ideal Torque Source/RConn1
  MOSFET4/LConn1 -- Simulink-PS Converter4/RConn1
  Ideal Torque Sensor/RConn2 -- " 1"/LConn1
  MOSFET1/LConn1 -- Simulink-PS Converter2/RConn1
  Permanent Magnet Synchronous Motor1/RConn1 -- Ideal Torque Sensor/LConn1
  Simulink-PS Converter6/RConn1 -- Controlled Voltage Source/RConn1
  Voltage Sensor1/RConn1 -- PS-Simulink Converter4/LConn1
  Simulink-PS Converter9/RConn1 -- Ideal Angular Velocity Source/RConn1
  Voltage Sensor/RConn1 -- PS-Simulink Converter2/LConn1
  MOSFET2/LConn1 -- Simulink-PS Converter1/RConn1
  Simulink-PS Converter5/RConn1 -- MOSFET3/LConn1
  " "/LConn1 -- Ideal Rotational Motion Sensor/RConn2
  Electrical Reference2/LConn1 -- Resistor/RConn1
  Current and Voltage Sensor (Three-Phase)/RConn3 -- Permanent Magnet Synchronous Motor1/LConn1

== system uz_codegen/DeadTime ==
  GateSignals : Inport
  Blanking Time : Subsystem  mask(Blanking Time){tb=T_dead}
      mask prompts: tb "Delay time:"
      mask help:
      | This block generates a blanking time for two-level inverter bridges so that the turn-on of one switch is delayed with respect to the turn-off of the other switch in the inverter leg.
      |
      | The input s is a switching function generated by a 2-level modulator. The values of the output s' are either 1, 0 or -1. If the input is a vector, the output is also a vector of the same width.
      mask Help: eval('plecs(''help'', ''blankingtime.html'')')
  Constant1 : Constant  Value=0.5
  Constant23 : Constant  Value=0.5
  Gain1 : Gain  Gain=0.5
  Gain5 : Gain  Gain=2
  Sum1 : Sum  Inputs=|++
  Sum6 : Sum  Inputs=|+-
  Out : Outport
  wires:
  Gain5/1 -> Blanking Time/1(s)
  Constant23/1 -> Sum6/2
  Sum6/1 -> Gain5/1
  Blanking Time/1(s') -> Gain1/1
  Constant1/1 -> Sum1/2
  Gain1/1 -> Sum1/1
  Sum1/1 -> Out/1
  GateSignals/1 -> Sum6/1

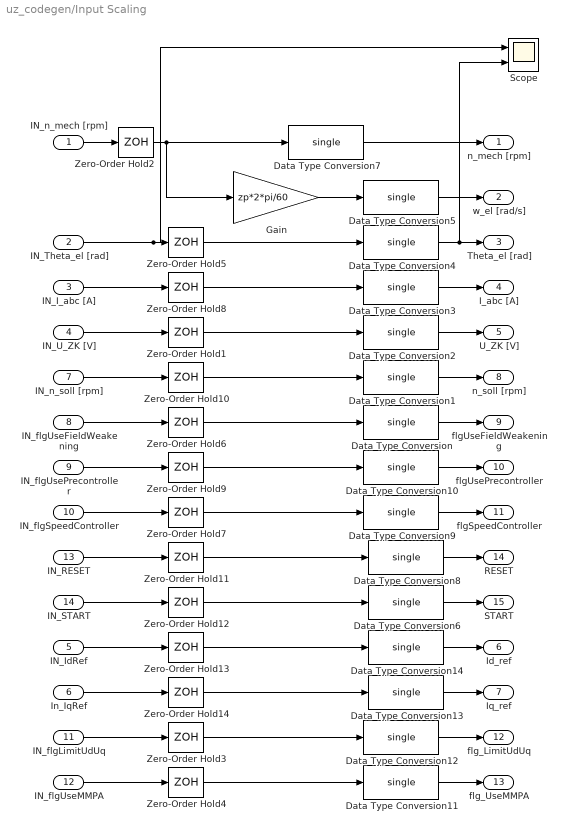
== system uz_codegen/Input Scaling ==
  IN_n_mech [rpm] : Inport
  IN_Theta_el [rad] : Inport  Port=2
  IN_I_abc [A] : Inport  Port=3
  IN_U_ZK [V] : Inport  Port=4
  IN_IdRef : Inport  Port=5
  In_IqRef : Inport  Port=6
  IN_n_soll [rpm] : Inport  Port=7
  IN_flgUseFieldWeakening : Inport  Port=8
  IN_flgUsePrecontroller : Inport  Port=9
  IN_flgSpeedController : Inport  Port=10
  IN_flgLimitUdUq : Inport  Port=11
  IN_flgUseMMPA : Inport  Port=12
  IN_RESET : Inport  Port=13
  IN_START : Inport  Port=14
  Data Type Conversion{,1..14} (15 alike) : DataTypeConversion  OutDataTypeStr=single
  Gain : Gain  Gain=zp*2*pi/60
  Scope : Scope  NumInputPorts=2
  Zero-Order Hold{1..14} (14 alike) : ZeroOrderHold  SampleTime=T_controller
  n_mech [rpm] : Outport
  w_el [rad/s] : Outport  Port=2
  Theta_el [rad] : Outport  Port=3
  I_abc [A] : Outport  Port=4
  U_ZK [V] : Outport  Port=5
  Id_ref : Outport  Port=6
  Iq_ref : Outport  Port=7
  n_soll [rpm] : Outport  Port=8
  flgUseFieldWeakening : Outport  Port=9
  flgUsePrecontroller : Outport  Port=10
  flgSpeedController : Outport  Port=11
  flg_LimitUdUq : Outport  Port=12
  flg_UseMMPA : Outport  Port=13
  RESET : Outport  Port=14
  START : Outport  Port=15
  wires:
  IN_Theta_el [rad]/1 -> Scope/1, Zero-Order Hold5/1
  IN_I_abc [A]/1 -> Zero-Order Hold8/1
  IN_n_mech [rpm]/1 -> Zero-Order Hold2/1
  Gain/1 -> Data Type Conversion5/1
  Zero-Order Hold5/1 -> Data Type Conversion4/1
  Zero-Order Hold8/1 -> Data Type Conversion3/1
  Zero-Order Hold1/1 -> Data Type Conversion2/1
  IN_U_ZK [V]/1 -> Zero-Order Hold1/1
  IN_n_soll [rpm]/1 -> Zero-Order Hold10/1
  Zero-Order Hold10/1 -> Data Type Conversion1/1
  Zero-Order Hold6/1 -> Data Type Conversion/1
  IN_flgUsePrecontroller/1 -> Zero-Order Hold9/1
  Zero-Order Hold9/1 -> Data Type Conversion10/1
  IN_flgUseFieldWeakening/1 -> Zero-Order Hold6/1
  IN_flgSpeedController/1 -> Zero-Order Hold7/1
  Zero-Order Hold7/1 -> Data Type Conversion9/1
  Zero-Order Hold2/1 -> Data Type Conversion7/1, Gain/1
  IN_RESET/1 -> Zero-Order Hold11/1
  Zero-Order Hold11/1 -> Data Type Conversion8/1
  IN_START/1 -> Zero-Order Hold12/1
  Zero-Order Hold12/1 -> Data Type Conversion6/1
  Zero-Order Hold13/1 -> Data Type Conversion14/1
  IN_IdRef/1 -> Zero-Order Hold13/1
  Zero-Order Hold14/1 -> Data Type Conversion13/1
  In_IqRef/1 -> Zero-Order Hold14/1
  IN_flgLimitUdUq/1 -> Zero-Order Hold3/1
  Zero-Order Hold3/1 -> Data Type Conversion12/1
  Zero-Order Hold4/1 -> Data Type Conversion11/1
  IN_flgUseMMPA/1 -> Zero-Order Hold4/1
  Data Type Conversion7/1 -> n_mech [rpm]/1
  Data Type Conversion5/1 -> w_el [rad/s]/1
  Data Type Conversion4/1 -> Scope/2, Theta_el [rad]/1
  Data Type Conversion3/1 -> I_abc [A]/1
  Data Type Conversion2/1 -> U_ZK [V]/1
  Data Type Conversion1/1 -> n_soll [rpm]/1
  Data Type Conversion/1 -> flgUseFieldWeakening/1
  Data Type Conversion10/1 -> flgUsePrecontroller/1
  Data Type Conversion9/1 -> flgSpeedController/1
  Data Type Conversion8/1 -> RESET/1
  Data Type Conversion6/1 -> START/1
  Data Type Conversion14/1 -> Id_ref/1
  Data Type Conversion13/1 -> Iq_ref/1
  Data Type Conversion12/1 -> flg_LimitUdUq/1
  Data Type Conversion11/1 -> flg_UseMMPA/1

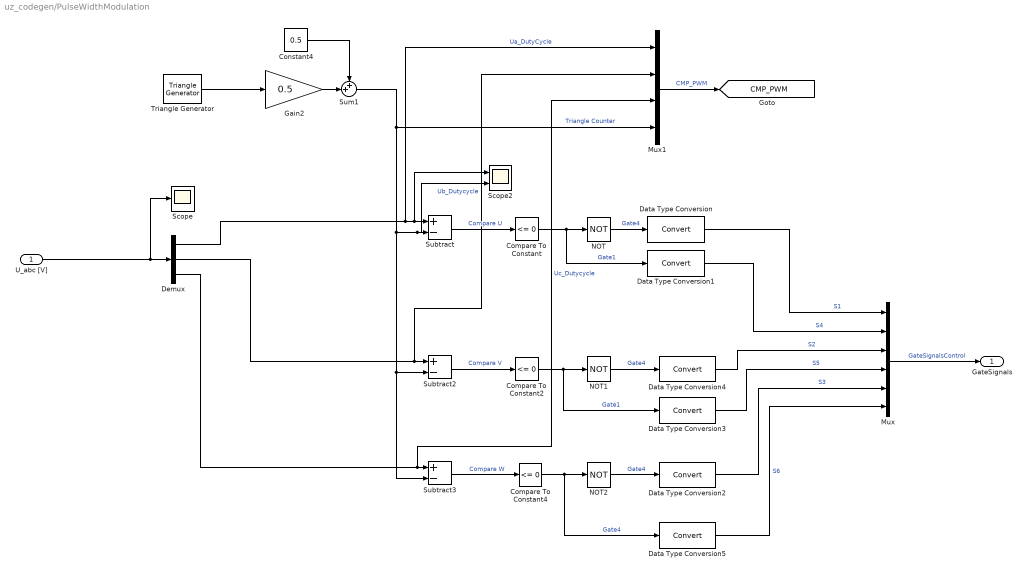
== system uz_codegen/PulseWidthModulation ==
  U_abc [V] : Inport
  Compare To Constant : simulink/Logic and Bit Operations/Compare To Constant  relop=<=  const=0  OutDataTypeStr=boolean
  Compare To Constant2 : simulink/Logic and Bit Operations/Compare To Constant  relop=<=  const=0  OutDataTypeStr=boolean
  Compare To Constant4 : simulink/Logic and Bit Operations/Compare To Constant  relop=<=  const=0  OutDataTypeStr=boolean
  Constant4 : Constant  Value=0.5
  Data Type Conversion{,1..5} (6 alike) : DataTypeConversion
  Demux : Demux  Outputs=3
  Gain2 : Gain  Gain=0.5
  Mux : Mux  Inputs=6
  Mux1 : Mux
  NOT : Logic  Operator=NOT  AllPortsSameDT=off  OutDataTypeStr=boolean
  NOT1 : Logic  Operator=NOT  IconShape=distinctive  AllPortsSameDT=off  OutDataTypeStr=boolean
  NOT2 : Logic  Operator=NOT  IconShape=distinctive  AllPortsSameDT=off  OutDataTypeStr=boolean
  Scope : Scope
  Scope2 : Scope  NumInputPorts=2
  Subtract : Sum  Inputs=+-
  Subtract2 : Sum  Inputs=+-
  Subtract3 : Sum  Inputs=+-
  Sum1 : Sum  Inputs=++|
  Triangle Generator : spsTriangleGeneratorLib/Triangle Generator  Freq=f_switchingInverter  Phase=0  Ts=0
  GateSignals : Outport
  tag scope: CMP_PWM=global
  wires:
  U_abc [V]/1 -> Scope/1, Demux/1
  Compare To Constant/1 -> Data Type Conversion1/1, NOT/1  "Gate1"
  Data Type Conversion1/1 -> Mux/2  "S4"
  Demux/1 -> Mux1/1, Scope2/1, Subtract/1  "Ua_DutyCycle"
  Data Type Conversion/1 -> Mux/1  "S1"
  Compare To Constant4/1 -> Data Type Conversion5/1, NOT2/1  "Gate4"
  Data Type Conversion4/1 -> Mux/3  "S2"
  Demux/2 -> Mux1/2, Subtract2/1  "Ub_Dutycycle"
  Subtract/1 -> Compare To Constant/1  "Compare U"
  Subtract3/1 -> Compare To Constant4/1  "Compare W"
  Demux/3 -> Mux1/3, Subtract3/1  "Uc_Dutycycle"
  Compare To Constant2/1 -> Data Type Conversion3/1, NOT1/1  "Gate1"
  Data Type Conversion5/1 -> Mux/6  "S6"
  Subtract2/1 -> Compare To Constant2/1  "Compare V"
  Data Type Conversion2/1 -> Mux/5  "S3"
  Data Type Conversion3/1 -> Mux/4  "S5"
  Constant4/1 -> Sum1/1
  Gain2/1 -> Sum1/2
  Triangle Generator/1 -> Gain2/1
  Sum1/1 -> Mux1/4, Scope2/2, Subtract/2, Subtract2/2, Subtract3/2  "Triangle Counter"
  Mux/1 -> GateSignals/1  "GateSignalsControl"
  NOT/1 -> Data Type Conversion/1  "Gate4"
  NOT1/1 -> Data Type Conversion4/1  "Gate4"
  NOT2/1 -> Data Type Conversion2/1  "Gate4"
  Mux1/1 -> [CMP_PWM]  "CMP_PWM"

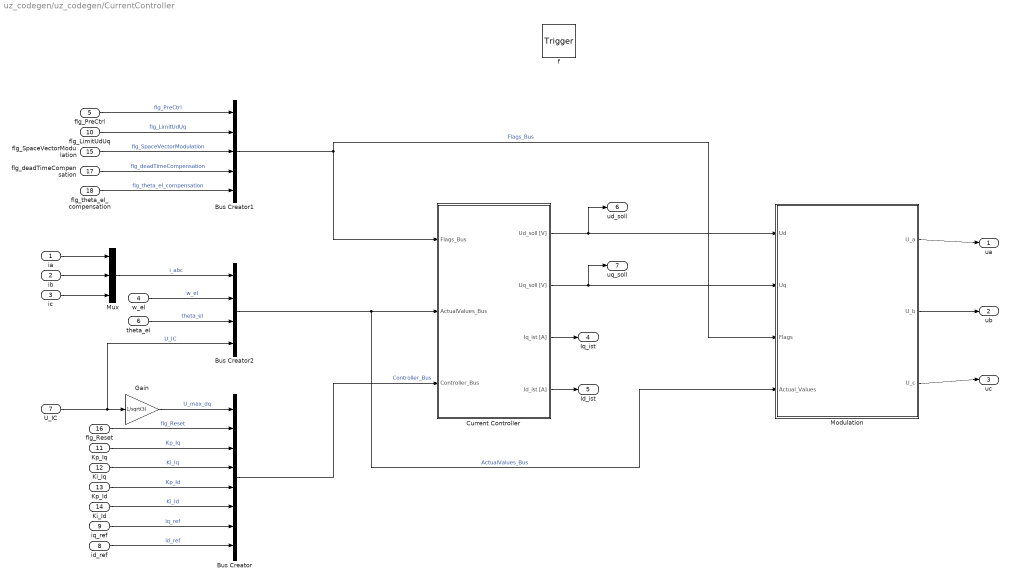
== system uz_codegen/uz_codegen/CurrentController ==
  ia : Inport  OutDataTypeStr=double  PortDimensions=1
  ib : Inport  Port=2  OutDataTypeStr=double  PortDimensions=1
  ic : Inport  Port=3  OutDataTypeStr=double  PortDimensions=1
  w_el : Inport  Port=4  OutDataTypeStr=double  PortDimensions=1
  flg_PreCtrl : Inport  Port=5  OutDataTypeStr=double  PortDimensions=1
  theta_el : Inport  Port=6  OutDataTypeStr=double  PortDimensions=1
  U_IC : Inport  Port=7  OutDataTypeStr=double  PortDimensions=1
  id_ref : Inport  Port=8  OutDataTypeStr=double  PortDimensions=1
  iq_ref : Inport  Port=9  OutDataTypeStr=double  PortDimensions=1
  flg_LimitUdUq : Inport  Port=10  OutDataTypeStr=double  PortDimensions=1
  Kp_Iq : Inport  Port=11  OutDataTypeStr=double  PortDimensions=1
  Ki_Iq : Inport  Port=12  OutDataTypeStr=double  PortDimensions=1
  Kp_Id : Inport  Port=13  OutDataTypeStr=double  PortDimensions=1
  Ki_Id : Inport  Port=14  OutDataTypeStr=double  PortDimensions=1
  flg_SpaceVectorModulation : Inport  Port=15  OutDataTypeStr=double  PortDimensions=1
  flg_Reset : Inport  Port=16  OutDataTypeStr=double  PortDimensions=1
  flg_deadTimeCompensation : Inport  Port=17  OutDataTypeStr=double  PortDimensions=1
  flg_theta_el_compensation : Inport  Port=18  OutDataTypeStr=double  PortDimensions=1
  f : TriggerPort  TriggerType=function-call  VariantControl=(inherit)
      settings: CopyFcn=Stateflow.SLINSF.SimulinkMan.removeBlockPreDeleteFcn  PreDeleteFcn=Stateflow.SLINSF.SimulinkMan.unsafePredeleteFcn
  Bus Creator : BusCreator  Inputs=8
  Bus Creator1 : BusCreator  Inputs=5
  Bus Creator2 : BusCreator  Inputs=4
  Current Controller : Subsystem
  Gain : Gain  Gain=1/sqrt(3)
  Modulation : Subsystem
  Mux : Mux  Inputs=3
  ua : Outport
  ub : Outport  Port=2
  uc : Outport  Port=3
  Iq_ist : Outport  Port=4
  Id_ist : Outport  Port=5
  ud_soll : Outport  Port=6
  uq_soll : Outport  Port=7
  wires:
  Current Controller/2(Uq_soll [V]) -> uq_soll/1, Modulation/2(Uq)
  U_IC/1 -> Gain/1, Bus Creator2/4  "U_IC"
  ib/1 -> Mux/2
  ia/1 -> Mux/1
  ic/1 -> Mux/3
  Current Controller/3(Iq_ist [A]) -> Iq_ist/1
  Current Controller/4(Id_ist [A]) -> Id_ist/1
  Current Controller/1(Ud_soll [V]) -> Modulation/1(Ud), ud_soll/1
  Gain/1 -> Bus Creator/1  "U_max_dq"
  flg_Reset/1 -> Bus Creator/2  "flg_Reset"
  Ki_Iq/1 -> Bus Creator/4  "Ki_Iq"
  Kp_Iq/1 -> Bus Creator/3  "Kp_Iq"
  Ki_Id/1 -> Bus Creator/6  "Ki_Id"
  Kp_Id/1 -> Bus Creator/5  "Kp_Id"
  Bus Creator/1 -> Current Controller/3(Controller_Bus)  "Controller_Bus"
  iq_ref/1 -> Bus Creator/7  "iq_ref"
  id_ref/1 -> Bus Creator/8  "id_ref"
  flg_deadTimeCompensation/1 -> Bus Creator1/4  "flg_deadTimeCompensation"
  flg_SpaceVectorModulation/1 -> Bus Creator1/3  "flg_SpaceVectorModulation"
  flg_LimitUdUq/1 -> Bus Creator1/2  "flg_LimitUdUq"
  flg_PreCtrl/1 -> Bus Creator1/1  "flg_PreCtrl"
  Bus Creator1/1 -> Modulation/3(Flags), Current Controller/1(Flags_Bus)  "Flags_Bus"
  Mux/1 -> Bus Creator2/1  "i_abc"
  w_el/1 -> Bus Creator2/2  "w_el"
  theta_el/1 -> Bus Creator2/3  "theta_el"
  Bus Creator2/1 -> Modulation/4(Actual_Values), Current Controller/2(ActualValues_Bus)  "ActualValues_Bus"
  Modulation/1(U_a) -> ua/1
  Modulation/2(U_b) -> ub/1
  Modulation/3(U_c) -> uc/1
  flg_theta_el_compensation/1 -> Bus Creator1/5  "flg_theta_el_compensation"

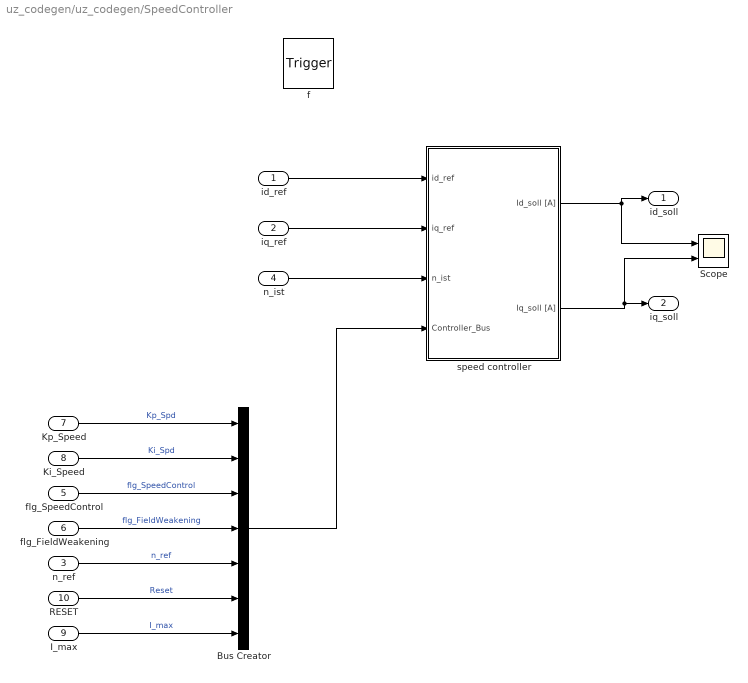
== system uz_codegen/uz_codegen/SpeedController ==
  id_ref : Inport  OutDataTypeStr=double  PortDimensions=1
  iq_ref : Inport  Port=2  OutDataTypeStr=double  PortDimensions=1
  n_ref : Inport  Port=3  OutDataTypeStr=double  PortDimensions=1
  n_ist : Inport  Port=4  OutDataTypeStr=double  PortDimensions=1
  flg_SpeedControl : Inport  Port=5  OutDataTypeStr=double  PortDimensions=1
  flg_FieldWeakening : Inport  Port=6  OutDataTypeStr=double  PortDimensions=1
  Kp_Speed : Inport  Port=7  OutDataTypeStr=double  PortDimensions=1
  Ki_Speed : Inport  Port=8  OutDataTypeStr=double  PortDimensions=1
  I_max : Inport  Port=9  OutDataTypeStr=double  PortDimensions=1
  RESET : Inport  Port=10  OutDataTypeStr=double  PortDimensions=1
  f : TriggerPort  TriggerType=function-call  VariantControl=(inherit)
      settings: CopyFcn=Stateflow.SLINSF.SimulinkMan.removeBlockPreDeleteFcn  PreDeleteFcn=Stateflow.SLINSF.SimulinkMan.unsafePredeleteFcn
  Bus Creator : BusCreator  Inputs=7
  Scope : Scope  NumInputPorts=2
  speed controller : Subsystem
  id_soll : Outport
  iq_soll : Outport  Port=2
  wires:
  n_ist/1 -> speed controller/3(n_ist)
  speed controller/1(Id_soll [A]) -> id_soll/1, Scope/1
  speed controller/2(Iq_soll [A]) -> Scope/2, iq_soll/1
  Kp_Speed/1 -> Bus Creator/1  "Kp_Spd"
  Ki_Speed/1 -> Bus Creator/2  "Ki_Spd"
  flg_SpeedControl/1 -> Bus Creator/3  "flg_SpeedControl"
  flg_FieldWeakening/1 -> Bus Creator/4  "flg_FieldWeakening"
  n_ref/1 -> Bus Creator/5  "n_ref"
  RESET/1 -> Bus Creator/6  "Reset"
  Bus Creator/1 -> speed controller/4(Controller_Bus)
  iq_ref/1 -> speed controller/2(iq_ref)
  id_ref/1 -> speed controller/1(id_ref)
  I_max/1 -> Bus Creator/7  "I_max"

== system uz_codegen/wrapto2pi ==
  Theta_raw : Inport
  Modulo by Constant : embmathops/Modulo by Constant  Denominator=2*pi  SimulateUsing=Code generation
      settings: SourceProductBaseCode=SL
  Theta_wrapped : Outport
  wires:
  Theta_raw/1 -> Modulo by Constant/1
  Modulo by Constant/1 -> Theta_wrapped/1
